simulink model "model"  (R2025b)
settings: Solver=VariableStepAuto  StartTime=0.0  StopTime=t_finish  FixedStep=dt1  RelTol=1e-5
values from neighbouring files (symbols this model uses):
  A = [0 1 0; 0 0 1; -1 -3 -2]    [code.m]
  A_u = [0 1; -1/4 0]    [code.m]
  Ad1 = expm(A*dt1)    [code.m]
  Ad1_u = expm(A_u*dt1)    [code.m]
  Ad2 = expm(A*dt2)    [code.m]
  Ad2_u = expm(A_u*dt2)    [code.m]
  b = [1; 1; 1]    [code.m]
  bd1 = inv(A)*(Ad1 - eye(rank(A)))*b    [code.m]
  bd2 = inv(A)*(Ad2 - eye(rank(A)))*b    [code.m]
  c = [1 1 1]    [code.m]
  c_u = [1 0]    [code.m]
  dt1 = 0.1    [code.m]
  dt2 = 0.01    [code.m]
  u_0 = [-pi/2; 0]    [code.m]
settings Model: Creator=shume  LastModifiedBy=user
settings RTWCC: GPUComputeCapability=3.5

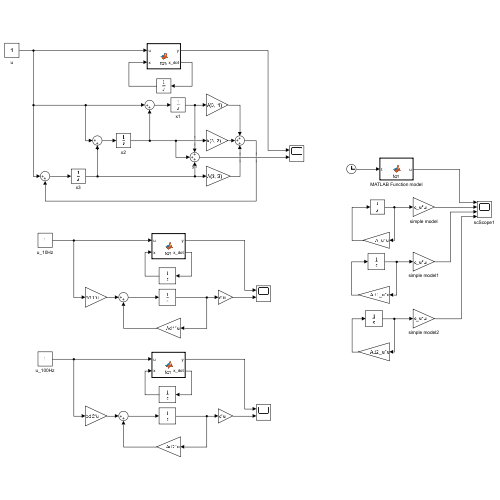
[thumbnail: Simulink's stored preview of the top-level diagram]
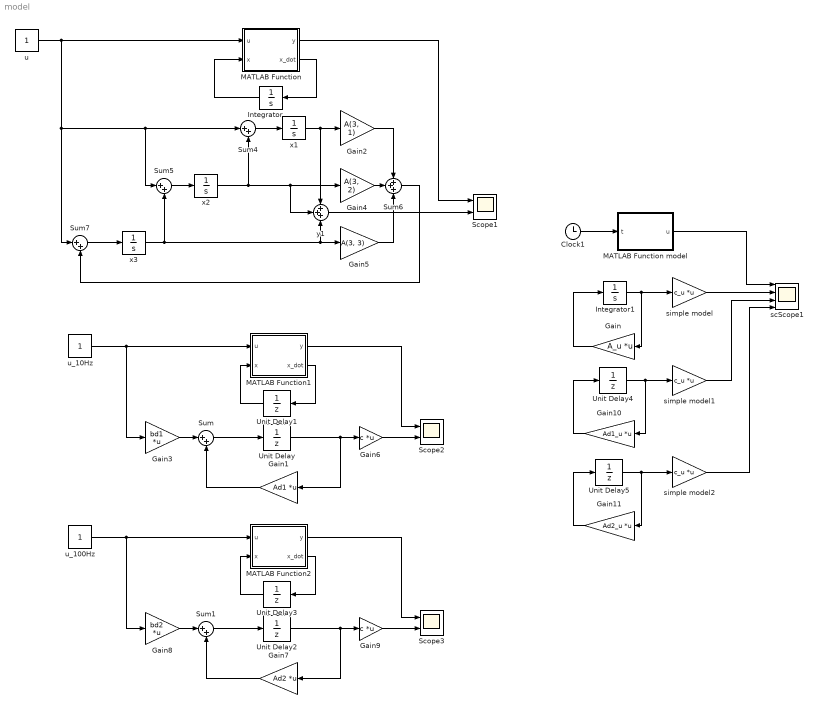
== system model ==
  Clock1 : Clock
  Gain : Gain  Gain=A_u  Multiplication=Matrix(K*u)
  Gain1 : Gain  Gain=Ad1  Multiplication=Matrix(K*u)
  Gain10 : Gain  Gain=Ad1_u  Multiplication=Matrix(K*u)
  Gain11 : Gain  Gain=Ad2_u  Multiplication=Matrix(K*u)
  Gain2 : Gain  Gain=A(3, 1)
  Gain3 : Gain  Gain=bd1  Multiplication=Matrix(K*u)
  Gain4 : Gain  Gain=A(3, 2)
  Gain5 : Gain  Gain=A(3, 3)
  Gain6 : Gain  Gain=c  Multiplication=Matrix(K*u)
  Gain7 : Gain  Gain=Ad2  Multiplication=Matrix(K*u)
  Gain8 : Gain  Gain=bd2  Multiplication=Matrix(K*u)
  Gain9 : Gain  Gain=c  Multiplication=Matrix(K*u)
  Integrator : Integrator  InitialCondition=[0; 0; 0]
  Integrator1 : Integrator  InitialCondition=u_0
  MATLAB Function : MATLAB Function  TreatAsAtomicUnit=on
  MATLAB Function model : MATLAB Function  TreatAsAtomicUnit=on
  MATLAB Function1 : MATLAB Function  TreatAsAtomicUnit=on
  MATLAB Function2 : MATLAB Function  TreatAsAtomicUnit=on
  Scope1 : Scope  NumInputPorts=2
      settings: ActiveDisplayYMinimum=-0.49213  ActiveDisplayYMaximum=4.42915  DataLoggingVariableName=ScopeData2
  Scope2 : Scope  NumInputPorts=2
      settings: ActiveDisplayYMinimum=-0.49212792009007972  ActiveDisplayYMaximum=4.4291512808107187
  Scope3 : Scope  NumInputPorts=2
      settings: ActiveDisplayYMinimum=-0.49212792009007972  ActiveDisplayYMaximum=4.4291512808107187  DataLoggingVariableName=ScopeData3
  Sum{,1,4..5,7} (5 alike) : Sum  Inputs=|++
  Sum6 : Sum  Inputs=+++
  Unit Delay : UnitDelay  SampleTime=dt1  HasFrameUpgradeWarning=on
  Unit Delay1 : UnitDelay  InitialCondition=[0; 0; 0]  SampleTime=dt1  HasFrameUpgradeWarning=on
  Unit Delay2 : UnitDelay  SampleTime=dt2  HasFrameUpgradeWarning=on
  Unit Delay3 : UnitDelay  InitialCondition=[0; 0; 0]  SampleTime=dt2  HasFrameUpgradeWarning=on
  Unit Delay4 : UnitDelay  InitialCondition=u_0  SampleTime=dt1  HasFrameUpgradeWarning=on
  Unit Delay5 : UnitDelay  InitialCondition=u_0  SampleTime=dt2  HasFrameUpgradeWarning=on
  scScope1 : Scope  NumInputPorts=4
      settings: ActiveDisplayYMinimum=0.781855833896284  ActiveDisplayYMaximum=0.81513383112355053  YLabel=u
  simple model : Gain  Gain=c_u  Multiplication=Matrix(K*u)
  simple model1 : Gain  Gain=c_u  Multiplication=Matrix(K*u)
  simple model2 : Gain  Gain=c_u  Multiplication=Matrix(K*u)
  u : Constant
  u_100Hz : Constant
  u_10Hz : Constant
  x1 : Integrator
  x2 : Integrator
  x3 : Integrator
  y1 : Sum  Inputs=+++
  wires:
  Integrator1/1 -> simple model/1, Gain/1
  Gain/1 -> Integrator1/1
  Clock1/1 -> MATLAB Function model/1(t)
  MATLAB Function model/1(u) -> scScope1/1
  simple model/1 -> scScope1/2
  MATLAB Function/2(x_dot) -> Integrator/1
  Integrator/1 -> MATLAB Function/2(x)
  u/1 -> MATLAB Function/1(u), Sum5/1, Sum4/1, Sum7/1
  Sum4/1 -> x1/1
  x2/1 -> y1/2, Gain4/1, Sum4/2
  Sum5/1 -> x2/1
  x3/1 -> y1/3, Gain5/1, Sum5/2
  x1/1 -> y1/1, Gain2/1
  Gain4/1 -> Sum6/2
  Gain5/1 -> Sum6/3
  Sum7/1 -> x3/1
  Sum6/1 -> Sum7/2
  y1/1 -> Scope1/2
  Gain2/1 -> Sum6/1
  MATLAB Function/1(y) -> Scope1/1
  MATLAB Function1/2(x_dot) -> Unit Delay1/1
  MATLAB Function1/1(y) -> Scope2/1
  Gain3/1 -> Sum/1
  Sum/1 -> Unit Delay/1
  Unit Delay/1 -> Gain6/1, Gain1/1
  Gain1/1 -> Sum/2
  Gain6/1 -> Scope2/2
  u_10Hz/1 -> Gain3/1, MATLAB Function1/1(u)
  Unit Delay1/1 -> MATLAB Function1/2(x)
  u_100Hz/1 -> Gain8/1, MATLAB Function2/1(u)
  Unit Delay3/1 -> MATLAB Function2/2(x)
  MATLAB Function2/2(x_dot) -> Unit Delay3/1
  Sum1/1 -> Unit Delay2/1
  Unit Delay2/1 -> Gain9/1, Gain7/1
  Gain9/1 -> Scope3/2
  Gain8/1 -> Sum1/1
  MATLAB Function2/1(y) -> Scope3/1
  Gain7/1 -> Sum1/2
  Gain10/1 -> Unit Delay4/1
  simple model1/1 -> scScope1/3
  simple model2/1 -> scScope1/4
  Gain11/1 -> Unit Delay5/1
  Unit Delay4/1 -> simple model1/1, Gain10/1
  Unit Delay5/1 -> Gain11/1, simple model2/1

== matlab function model/MATLAB Function model ==
  data: t input; u output
function u = fcn(t)

u = pi/2*cos(-0.5*t + pi);

== matlab function model/MATLAB Function ==
  data: y output; u input; x input; x_dot output; A parameter; b parameter; c parameter
function [y, x_dot] = fcn(u, x, A, b, c)

A = [0 1 0; 0 0 1; -1 -3 -2]; b = [1; 1; 1];

x_dot = A*x+b*u;
y = c*x;

== matlab function model/MATLAB Function1 ==
  data: y output; u input; x input; x_dot output; Ad1 parameter; bd1 parameter; c parameter
function [y, x_dot] = fcn(u, x, Ad1, bd1, c)

x_dot = Ad1*x+bd1*u;
y = c*x;

== matlab function model/MATLAB Function2 ==
  data: y output; u input; x input; x_dot output; Ad2 parameter; bd2 parameter; c parameter
function [y, x_dot] = fcn(u, x, Ad2, bd2, c)

x_dot = Ad2*x+bd2*u;
y = c*x;
